simulink model "signalModification"  (R2024a)
settings: Solver=VariableStepAuto  StartTime=0.0  StopTime=20  RelTol=1e-3
settings Model: Creator=hsllo  LastModifiedBy=hsllo

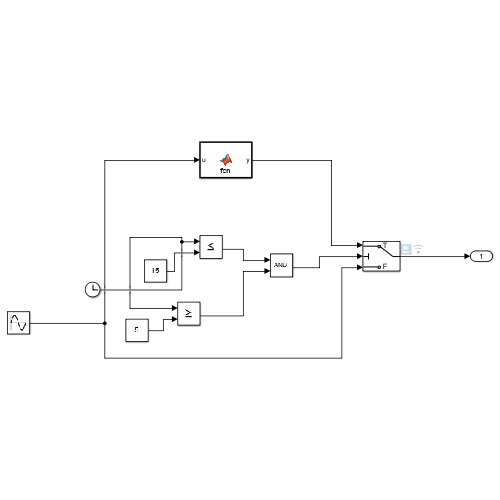
[thumbnail: Simulink's stored preview of the top-level diagram]
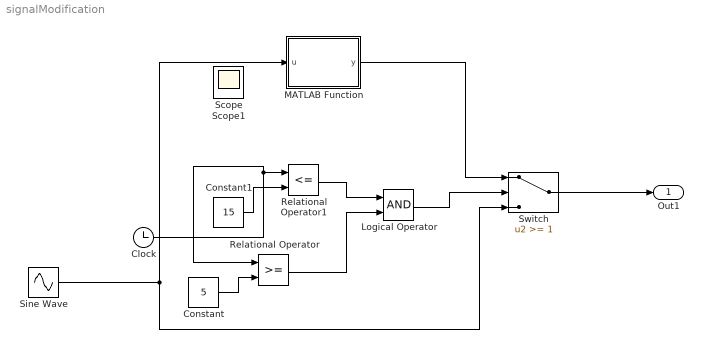
== system signalModification ==
  Clock : Clock
  Constant : Constant  Value=5
  Constant1 : Constant  Value=15
  Logical Operator : Logic  AllPortsSameDT=off  OutDataTypeStr=boolean
  MATLAB Function : MATLAB Function  TreatAsAtomicUnit=on
  Relational Operator : RelationalOperator  OutDataTypeStr=boolean  RndMeth=Simplest  InputSameDT=off
  Relational Operator1 : RelationalOperator  Operator=<=  OutDataTypeStr=boolean  RndMeth=Simplest  InputSameDT=off
  Sine Wave : Sin  SampleTime=0
  Switch : Switch  Threshold=1  SaturateOnIntegerOverflow=off  InputSameDT=off
  Out1 : Outport
  Scope : Scope
  Scope1 : Scope
  wires:
  Sine Wave/1 -> Switch/3, MATLAB Function/1(u)
  MATLAB Function/1(y) -> Switch/1
  Switch/1 -> Out1/1
  Constant/1 -> Relational Operator/2
  Clock/1 -> Relational Operator/1, Relational Operator1/1
  Constant1/1 -> Relational Operator1/2
  Relational Operator1/1 -> Logical Operator/1
  Relational Operator/1 -> Logical Operator/2
  Logical Operator/1 -> Switch/2

== matlab function signalModification/MATLAB Function ==
  data: u input; y output
function y = fcn(u)
    
    tempSignal = u;
    tempSignal1=tempSignal*10+20*normrnd(0,5);
    % tempSignal2=0;
    % cTime = getCurrentTime('test0718_01');
    % if(cTime>10)
    %     tempSignal2 = tempSignal1;
    % else
    %     tempSignal1 = tempSignal;
    % end
y = tempSignal1;
